simulink subsystem "three_way_valve"  (R2024b)
settings: Solver=VariableStepAuto  StartTime=0.0  StopTime=10.0  RelTol=1e-3
model mask{unknown_m=m_1, unknown_T=T_1}
  mask prompts: unknown_m "Mass flow"; unknown_T "Temperature"
settings Model: Creator=nerotb  LastModifiedBy=nerotb

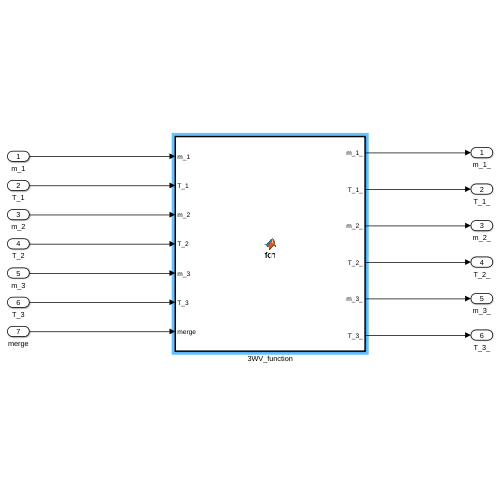
[thumbnail: Simulink's stored preview of the top-level diagram]
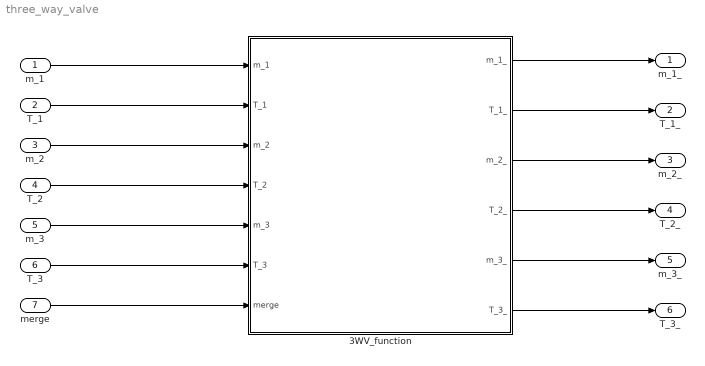
== system three_way_valve ==
  m_1 : Inport
  T_1 : Inport  Port=2
  m_2 : Inport  Port=3
  T_2 : Inport  Port=4
  m_3 : Inport  Port=5
  T_3 : Inport  Port=6
  merge : Inport  Port=7
  3WV_function : MATLAB Function  TreatAsAtomicUnit=on
  m_1_ : Outport
  T_1_ : Outport  Port=2
  m_2_ : Outport  Port=3
  T_2_ : Outport  Port=4
  m_3_ : Outport  Port=5
  T_3_ : Outport  Port=6
  wires:
  m_1/1 -> 3WV_function/1(m_1)
  T_1/1 -> 3WV_function/2(T_1)
  m_2/1 -> 3WV_function/3(m_2)
  T_2/1 -> 3WV_function/4(T_2)
  m_3/1 -> 3WV_function/5(m_3)
  T_3/1 -> 3WV_function/6(T_3)
  3WV_function/1(m_1_) -> m_1_/1
  3WV_function/2(T_1_) -> T_1_/1
  3WV_function/3(m_2_) -> m_2_/1
  3WV_function/4(T_2_) -> T_2_/1
  3WV_function/5(m_3_) -> m_3_/1
  3WV_function/6(T_3_) -> T_3_/1
  merge/1 -> 3WV_function/7(merge)

== matlab function three_way_valve/3WV_function ==
  data: m_1 input size=1; m_1_ output size=1; T_1 input size=1; m_2 input size=1; T_2 input size=1; m_3 input size=1; T_3 input size=1; T_1_ output size=1; m_2_ output size=1; T_2_ output size=1; m_3_ output size=1; T_3_ output size=1; merge input; unknown_m parameter size=1; unknown_T parameter size=1
function [m_1_, T_1_, m_2_, T_2_, m_3_, T_3_] = fcn(m_1, T_1, m_2, T_2, m_3, T_3, merge, unknown_m, unknown_T)
%% Summary: 
% This function models a generic 3-ways valve that can be used in two modes:
% - merge == 1: merging:               flow 1 (entering) is mixed with flow 2 (entering) to define flow 3 (exiting). 
% - merge == 0: diverging:             flow 1 (entering) defines flow 2 (exiting) and flow 3 (exiting). 
%
%% How to:
% 1. All input ports must be connected, 
% except for the two values (one temperature, one mass flow) to be determined which are specified in the component mask.
% 2. All 3 mass flows and 3 temperatures are available as outputs, with
% same values than input if specified
% identique à l'entrée lorsqu'elle est spécifiée
%
%% Conditions:
% - mass flow are non negative, i.e. >= 0
% - mass balance is conserved so basic inequalities must be verified
%
%   Call won't stop in case these hypothesis are not respected but some
%   values will be replaced
%
%% Hypothesis:
% - Equal Cp for all flows
%
%% Particular cases of the merging mode
% - if one of the entering flow has a null mass flow but unknown temperature (=to be determined),
% then this temperature is defined as the one of the other entering mass flow
% - If the exiting flow as a null mass flow but unknown temperature (=to be determined), 
% then this temperature is defined as the mean of entering temperatures

if m_1 < 0
    sprintf('3-way valve: m_1 < 0 (m_1=%1.2e), used value is m_1=0\n', m_1);
    m_1 = 0;
end

if m_2 < 0
    sprintf('3-way valve: m_2 < 0 (m_2=%1.2e), used value is m_2=0\n', m_2);
    m_2 = 0;
end

if m_3 < 0
    sprintf('3-way valve: m_3 < 0 (m_3=%1.2e), used value is m_3=0\n', m_3);
    m_3 = 0;
end


m_1_ = 1000;
m_2_ = 1000;
m_3_ = 1000;
T_1_ = 1000;
T_2_ = 1000;
T_3_ = 1000;

if merge
    % mass flow balance: m_1 + m_2 = m_3
    switch unknown_m
    case 1   % m_1 unknown
        if m_3 < m_2
            sprintf('3-way valve: m_3 (%1.2e) < m_2 (%1.2e), used value is m_2=m_3\n', m_3, m_2);
            m_2 = m_3;
        end
        m_2_ = m_2;
        m_3_ = m_3;
        m_1_ = m_3_ - m_2_; 
        
    case 2   % m_2 unknown
        if m_3 < m_1
            sprintf('3-way valve: m_3 (%1.2e) < m_1 (%1.2e), used value is m_1=m_3\n', m_3, m_1);
            m_1 = m_3;
        end
        m_1_ = m_1;
        m_3_ = m_3;
        m_2_ = m_3_ - m_1_;
    case 3   % m_3 unknown
        m_1_ = m_1;
        m_2_ = m_2;
        m_3_ = m_1_ + m_2_;
    end 

    % energy balance: m_1 * T_1 + m_2 * T_2 = m_3 * T_3
    switch unknown_T
        case 1   % T_1 unknown
            if m_1_ == 0   
                if T_2 ~= T_3
                    sprintf('3-way valve: T_2 (%2.1f) != T_3 (%2.1f), used value is T_2=T_3\n', T_2, T_3);
                    T_2 = T_3;
                end
                T_2_ = T_2;
                T_3_ = T_3;
                T_1_ = T_2; % non physical hypothesis
            else
                T_2_ = T_2;
                T_3_ = T_3;
                T_1_  = (m_3_ * T_3_ - m_2_ * T_2_ ) / m_1_;
            end
        
        case 2   % T_2 unknown
            if m_2_ == 0   
                if T_1 ~= T_3
                    sprintf('3-way valve: T_1 (%2.1f) != T_3 (%2.1f), used value is T_1=T_3\n', T_1, T_3);
                    T_1 = T_3;
                end

                T_1_ = T_1;
                T_3_ = T_3;
                T_2_ = T_1; % non physical hypothesis
            else
                T_1_ = T_1;
                T_3_ = T_3;
                T_2_  = (m_3_ * T_3_ - m_1_ * T_1_ ) / m_2_;
            end
        case 3   % T_3 unknown
            if m_3_ == 0   
                T_1_ = T_1;
                T_2_ = T_2;
                T_3_ = (T_1_ + T_2_) / 2; % non physical hypothesis
            else
                T_1_ = T_1;
                T_2_ = T_2;
                T_3_  = (m_1_ * T_1_ + m_2_ * T_2_ ) / m_3_;
            end
        end 


else % diverging
    % mass flow balance: m_1 = m_2 + m_3
    switch unknown_m
    case 1   % m_1 unknown
        m_2_ = m_2;
        m_3_ = m_3;
        m_1_ = m_2_ + m_3_; 
        
    case 2   % m_2 unknown
        if m_1 < m_3
            sprintf('3-way valve: m_1 (%1.2e) < m_3 (%1.2e), used value is m_3=m_1\n', m_1, m_3);
            m_3 = m_1;
        end
        m_1_ = m_1;
        m_3_ = m_3;
        m_2_ = m_1_ - m_3_;
    case 3   % m_3 unknown
        if m_1 < m_2
            sprintf('3-way valve: m_1 (%1.2e) < m_2 (%1.2e), used value is m_2=m_1\n', m_1, m_2);
            m_2 = m_1;
        end
        m_1_ = m_1;
        m_2_ = m_2;
        m_3_ = m_1_ - m_2_;
    end 

    % energy balance: T_1 = T_2 = T_3
    switch unknown_T
    case 1   % T_1 unknown
        if T_2 ~= T_3
            sprintf('3-way valve: T_2 (%2.1f) != T_3 (%2.1f), used value is T_2=T_3\n', T_2, T_3);
            T_2 = T_3;
        end
        T_2_ = T_2;
        T_3_ = T_3;
        T_1_ = T_2_;
        
    case 2   % T_2 unknown
        if T_1 ~= T_3
            sprintf('3-way valve: T_1 (%2.1f) != T_3 (%2.1f), used value is T_1=T_3\n', T_1, T_3);
            T_1 = T_3;
        end
        T_1_ = T_1;
        T_3_ = T_3;
        T_2_ = T_1_;
    case 3   % T_3 unknown
        if T_1 ~= T_2
            sprintf('3-way valve: T_1 (%2.1f) != T_2 (%2.1f), used value is T_1=T_2\n', T_1, T_2);
            T_1 = T_2;
        end
        T_1_ = T_1;
        T_2_ = T_2;
        T_3_ = T_1_;
    end 


end

end
